simulink model "ODE_Fucn1"  (R2020a)
settings: Solver=ode4  StartTime=ts  StopTime=tf  FixedStep=dt  RelTol=1e-3
values from neighbouring files (symbols this model uses):
  A = [ 0 1; -1 -2]    [my_main.m]
  B = [ 0; 1]    [my_main.m]
  c = 1    [my_main.m]
  ini = [2;2]    [my_main.m]
  k = 1    [my_main.m]
settings Model: Creator=TA  LastModifiedBy=TA

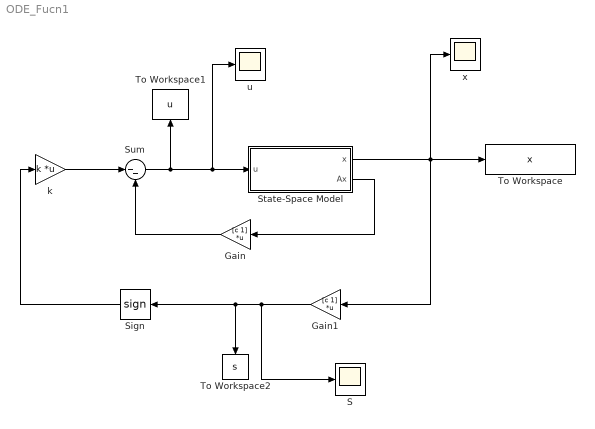
== system ODE_Fucn1 ==
  Gain : Gain  Gain=[c 1]  Multiplication=Matrix(K*u) (u vector)
  Gain1 : Gain  Gain=[c 1]  Multiplication=Matrix(K*u) (u vector)
  S : Scope
  Sign : Signum
  State-Space Model : Subsystem
  Sum : Sum  Inputs=|--
  To Workspace : ToWorkspace  VariableName=x  SampleTime=-1
  To Workspace1 : ToWorkspace  VariableName=u  SampleTime=-1
  To Workspace2 : ToWorkspace  VariableName=s  SampleTime=-1
  k : Gain  Gain=k  Multiplication=Matrix(K*u)
  u : Scope
  x : Scope
  wires:
  State-Space Model/2(Ax) -> Gain/1
  Gain/1 -> Sum/2
  Sum/1 -> u/1, State-Space Model/1(u), To Workspace1/1
  k/1 -> Sum/1
  Gain1/1 -> S/1, To Workspace2/1, Sign/1
  Sign/1 -> k/1
  State-Space Model/1(x) -> x/1, Gain1/1, To Workspace/1

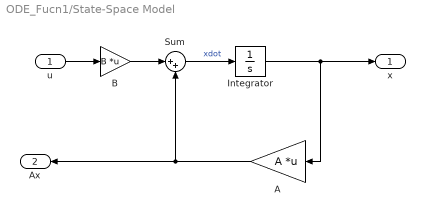
== system ODE_Fucn1/State-Space Model ==
  u : Inport
  A : Gain  Gain=A  Multiplication=Matrix(K*u) (u vector)
  B : Gain  Gain=B  Multiplication=Matrix(K*u) (u vector)
  Integrator : Integrator  InitialCondition=ini
  Sum : Sum  Inputs=|++
  x : Outport
  Ax : Outport  Port=2
  wires:
  u/1 -> B/1
  B/1 -> Sum/1
  Sum/1 -> Integrator/1  "xdot"
  Integrator/1 -> A/1, x/1
  A/1 -> Ax/1, Sum/2
